simulink model "Twist"  (R2018b)
settings: Solver=VariableStepAuto  StartTime=0.0  StopTime=10.0  RelTol=1e-3
values from neighbouring files (symbols this model uses):
  rotorInertia = 9.8946e-06    [nonLinearSim.m]
undefined symbols (not defined in the file or in its folder): sigbuilder_block
libraries: fl_lib x6, nesl_utility x5, elec_lib x3, cstblocks x1, sdl_lib x1
settings Model: Creator=Mark Sherstan  LastModifiedBy=Mark Sherstan

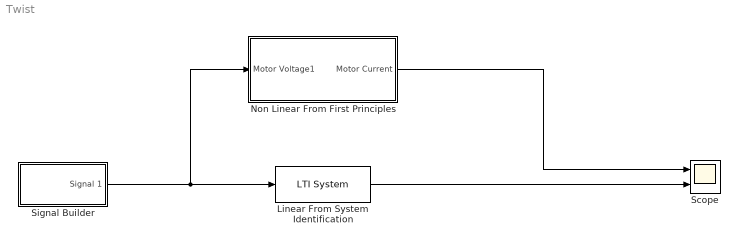
== system Twist ==
  Linear From System Identification : cstblocks/LTI System  sys=tf1  IC=[]
  Non Linear From First Principles : Subsystem
  Scope : Scope  NumInputPorts=2
  Signal Builder : Subsystem  Tag=STV Subsys  LoadFcn=sigbuilder_block('load');  StartFcn=sigbuilder_block('start');  StopFcn=sigbuilder_block('stop');  ClipboardFcn=sigbuilder_block('clipboard');  mask(Sigbuilder block){tuvar=[0:10]}
      mask help: Simulink:masks:SigbuilderBlock_MD
      mask init:
      | if ~strcmp(get_param(bdroot(gcbh),'SimulationStatus'),'stopped') tuvar = sigbuilder_block('maskInit'); end
      settings: CopyFcn=sigbuilder_block('copy');  DeleteFcn=sigbuilder_block('delete');  ModelCloseFcn=sigbuilder_block('modelClose');  PreSaveFcn=sigbuilder_block('preSave');  PauseFcn=sigbuilder_block('pause');  ContinueFcn=sigbuilder_block('continue');  NameChangeFcn=sigbuilder_block('namechange');  OpenFcn=sigbuilder_block('open',[437.6 199.2 550.4 400 ]);  CloseFcn=sigbuilder_block('close');
      mask Display: plot(0, 0, 100, 100,[2, 2, 32, 32, 2], [68, 8, 8, 68, 68],[32, 2], [38, 38], [32, 19, 2],[53, 60, 44], [32, 17, 17, 2],[16, 16, 31, 31]);txt = getActiveGroup(gcbh);text(2, 100, txt,'verticalAlignment', 'top');
  wires:
  Signal Builder/1(Signal 1) -> Non Linear From First Principles/1(Motor Voltage1), Linear From System Identification/1
  Linear From System Identification/1 -> Scope/2
  Non Linear From First Principles/1(Motor Current) -> Scope/1

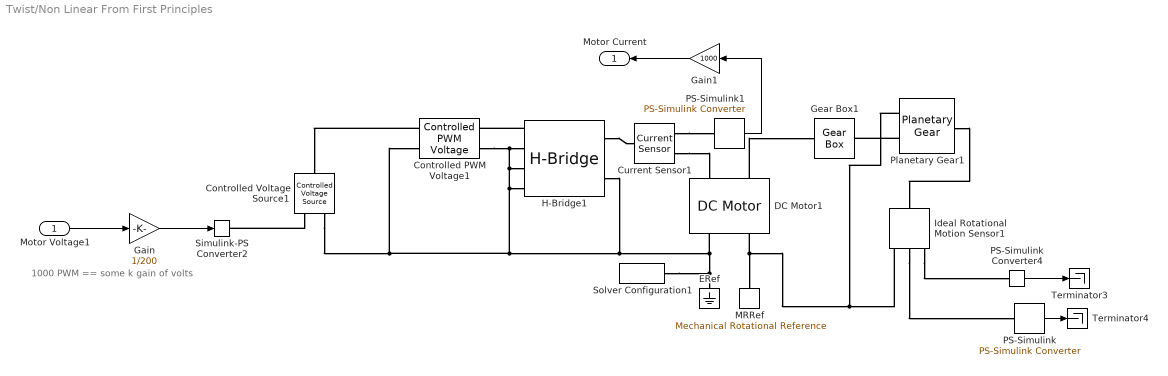
== system Twist/Non Linear From First Principles ==
  note: 1000 PWM == some k gain of volts
  Motor Voltage1 : Inport
  Controlled PWM Voltage1 : elec_lib/Actuators & Drivers/Drivers/Controlled PWM Voltage  F=4000 Hz  TD=0 s  pulse_width_offset=0 s  pulse_min=0 s  Vmin=0 V  Vmax=5 V  Vm=5 V  pwm_or_av=2  event_type=1  sample_time=1e-6 s  u_min=0  u_max=1
      settings: SourceProductName=Simscape Electronics  SourceProductBaseCode=SN
  Controlled Voltage Source1 : fl_lib/Electrical/Electrical Sources/Controlled Voltage Source
  Current Sensor1 : fl_lib/Electrical/Electrical Sensors/Current Sensor
      settings: SourceProductName=Foundation Library
  DC Motor1 : elec_lib/Actuators & Drivers/Rotational Actuators/DC Motor  parameterization=2  Ra=3.38 Ohm  La=armatureInduc H  emf_or_torque=1  Kv=0.029 V/(rad/s)  Ki=6.876e-04 N*m/A  T_stall=stallTorque N*m  w_max=noLoadSpeed rpm  w_rated=2500 rpm  P_rated=10 W  V_rated=RatedV V  J=rotorInertia kg*m^2  lam_param=2  lam=0.5e-5 N*m/(rad/s)  i_noload=noLoadCurrent A  V_i_noload=supply4noLoadCurrent V  speed0=0 rpm  alpha=0.00393 1/K  Tmeas=25 degC  thermal_mass=100 J/K  initial_temperature=25 degC
  ERef : fl_lib/Electrical/Electrical Elements/Electrical Reference
      settings: SourceProductName=Foundation Library
  Gain : Gain  Gain=1/200
  Gain1 : Gain  Gain=1000
  Gear Box1 : fl_lib/Mechanical/Mechanisms/Gear Box  ratio=2  t_in_specify=off  t_in_priority=None  t_in=0 N*m  t_in_nominal_specify=off  t_in_nominal_unit=N*m  t_in_nominal_value=1  t_out_specify=off  t_out_priority=None  t_out=0 N*m  t_out_nominal_specify=off  t_out_nominal_unit=N*m  t_out_nominal_value=1
  H-Bridge1 : elec_lib/Actuators & Drivers/Drivers/H-Bridge  Venable=2.5 V  Vmax=5 V  Vreverse=2.5 V  Vbrake=2.5 V  Vm=12 V  pwm_or_av=2  discontinuous=0  freewheeling_mode=1  freewheeling_mode_disc=1  Ron=0.1 Ohm  Don=0.1 Ohm  Rload=3.38+0.1 Ohm  Lload=1e-5 H  F=4 kHz  thermal_mass=100 J/K  initial_temperature=298.15 K  Ron2=0.1 Ohm  Don2=0.05 Ohm  Tmeas=298.15 K  Tmeas2=398.15 K
      settings: SourceProductName=Simscape Electronics  SourceProductBaseCode=SN
  Ideal Rotational Motion Sensor1 : fl_lib/Mechanical/Mechanical Sensors/Ideal Rotational Motion Sensor  offset=0 deg
      settings: SourceProductName=Foundation Library
  MRRef : fl_lib/Mechanical/Rotational Elements/Mechanical Rotational Reference
      settings: SourceProductName=Foundation Library
  PS-Simulink : nesl_utility/PS-Simulink Converter  PhysicalDomain=network_engine_domain  SubClassName=ps_output  LeftPortType=input  RightPortType=output  PseudoPeriodic=off  Frequencies=[]  Unit=rpm  AffineConversion=off
  PS-Simulink Converter4 : nesl_utility/PS-Simulink Converter  PhysicalDomain=network_engine_domain  SubClassName=ps_output  LeftPortType=input  RightPortType=output  PseudoPeriodic=off  Frequencies=[]  Unit=1  AffineConversion=off
  PS-Simulink1 : nesl_utility/PS-Simulink Converter  PhysicalDomain=network_engine_domain  SubClassName=ps_output  LeftPortType=input  RightPortType=output  PseudoPeriodic=off  Frequencies=[]  Unit=A  AffineConversion=off
  Planetary Gear1 : sdl_lib/Gears/Planetary Gear  rs_ratio=3.5  friction_model=1  efficiency=[.96, .98]  mu_visc=[0, 0] N*m/(rad/s)  pwr_thr=[.001, .001] W  planet_inertia=0 kg*m^2  temperature_TLU=[280, 300, 320] K  efficiency_sp_TLU=[.95, .9, .85]  efficiency_rp_TLU=[.95, .9, .85]  thermal_mass=50 J/K  T_init=300 K
      settings: SourceProductName=Simscape Driveline  SourceProductBaseCode=LD
  Simulink-PS Converter2 : nesl_utility/Simulink-PS Converter  PhysicalDomain=network_engine_domain  SubClassName=ps_input  LeftPortType=input  RightPortType=output  PseudoPeriodic=off  Frequencies=[]  NoiseDistribution=none  NoiseParameters=[]  Unit=1  AffineConversion=off  FilteringAndDerivatives=provide  SimscapeFilterOrder=1  InputFilterTimeConstant=0.001  UdotUserProvided=0
  Solver Configuration1 : nesl_utility/Solver Configuration  PhysicalDomain=network_engine_domain  SubClassName=solver  LeftPortType=input  RightPortType=generic  Tones=[]  Harmonics=[]  SimulateNoise=off  Profile=off  UseLocalSampling=off  EnableSwitchedLinearOptims=on  FrequencyDomain=off  UseCCode=off  RelTol=0.001  AbsTol=1e-06  MinStep=1e-09  ToWorkspace=off  RevertToSquareIcSolve=off  NumHomotopyIterations=100  PhasorMode=off  PhasorModeNumHarmonics=1  DoDC=off  ResidualTolerance=1e-9  UseLocalSolver=off  LocalSolverChoice=NE_BACKWARD_EULER_ADVANCER  LocalSolverSampleTime=.001  DoFixedCost=off  MaxNonlinIter=3  MaxModeIter=2  LinearAlgebra=auto  EquationFormulation=NE_TIME_EF  DelaysMemoryBudget=1024  AutomaticFiltering=on  FilteringTimeConstant=0.001  PartitionStorageMethod=AS_NEEDED  PartitionMemoryBudget=1024
  Terminator3 : Terminator
  Terminator4 : Terminator
  Motor Current : Outport
  wires:
  Motor Voltage1/1 -> Gain/1
  Gain/1 -> Simulink-PS Converter2/1
  PS-Simulink Converter4/1 -> Terminator3/1
  PS-Simulink/1 -> Terminator4/1
  Gain1/1 -> Motor Current/1
  PS-Simulink1/1 -> Gain1/1
  connections:
  ERef/LConn1 -- Controlled Voltage Source1/RConn2 -- Controlled PWM Voltage1/LConn2 -- H-Bridge1/LConn2 -- Controlled PWM Voltage1/RConn2 -- H-Bridge1/LConn3 -- H-Bridge1/LConn4 -- H-Bridge1/RConn2 -- DC Motor1/RConn1 -- Solver Configuration1/RConn1
  Ideal Rotational Motion Sensor1/RConn1 -- Planetary Gear1/RConn1 -- DC Motor1/RConn2 -- MRRef/LConn1
  Controlled PWM Voltage1/LConn1 -- Controlled Voltage Source1/LConn1
  Ideal Rotational Motion Sensor1/RConn2 -- PS-Simulink/LConn1
  Current Sensor1/RConn2 -- DC Motor1/LConn1
  Ideal Rotational Motion Sensor1/RConn3 -- PS-Simulink Converter4/LConn1
  H-Bridge1/RConn1 -- Current Sensor1/LConn1
  Planetary Gear1/RConn2 -- Gear Box1/RConn1
  Current Sensor1/RConn1 -- PS-Simulink1/LConn1
  DC Motor1/LConn2 -- Gear Box1/LConn1
  Planetary Gear1/LConn1 -- Ideal Rotational Motion Sensor1/LConn1
  H-Bridge1/LConn1 -- Controlled PWM Voltage1/RConn1
  Controlled Voltage Source1/RConn1 -- Simulink-PS Converter2/RConn1

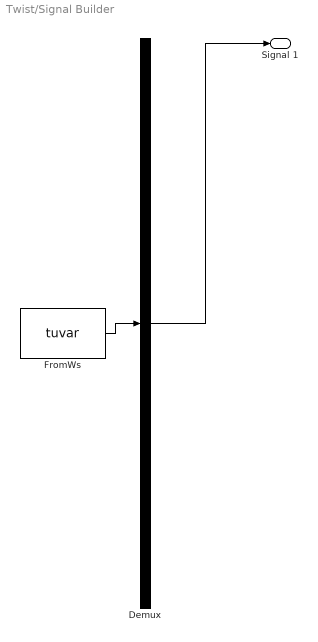
== system Twist/Signal Builder ==
  Demux : Demux  Tag=STV Demux  Outputs=1
  FromWs : FromWorkspace  Tag=STV FromWs  VariableName=tuvar  SampleTime=0
      SigBuilderData=|
      | common.afterFinalStr = 'Extrapolate'
      | common.sampleTime = 0
      | dataSet.timeRange = [0 10]
      | dataSet.name = 'Group 1'
      | sbobj.Groups.Name = 'Group 1'
      | sbobj.Groups.Signals.Name = 'Signal 1'
      | sbobj.Groups.Signals.XData = [0 2.98 2.98 7 7 10]
      | sbobj.Groups.Signals.YData = [0 0 1000 1000 500 31]
  Signal 1 : Outport  Tag=STV Outport
  wires:
  Demux/1 -> Signal 1/1
  FromWs/1 -> Demux/1
